simulink model "lab3_step3"  (R2019b)
settings: Solver=VariableStepAuto  StartTime=0.0  StopTime=stop_time  RelTol=1e-3
InitFcn:
  | %Read in the audio file
  | [input_wav_signal, Fs_in] = audioread('acoustic.wav');
  | % Fs_in = 11025 and we need to convert this to Fs = 48k
  | 
  | % COnvert the Sampling rate to 48 kHz
  | signal = resample(input_wav_signal, 48000, 11025);
  | Fs = 48000; % This is out desired sample rate that we converted to
  | Ts = 1/Fs;    % and the associated sample period.
  | 
  | % Put signal into a timeseries format
  | timevals = [0:length(signal)-1]*Ts;
  | input_signal = timeseries(signal,timevals);
  | 
  | % Set the simulation stop time
  | stop_time = length(signal) * Ts; % set the simulation time the same length as the input signal
  | 
  | 
  | % Fixed-point precision we want the signal converted to.
  | W_bits = 32;
  | F_bits = 28;
  | 
  | max_reset_Nsamples = 1024*16 % should be a power of 2
  | max_reset_Nbits = ceil (log2 (max_reset_Nsamples));
StopFcn:
  | y_out = output_signal.Data(:);
  | plot(y_out)
  | soundsc(y_out,Fs)
undefined symbols (not defined in the file): magnitude
libraries: simulink x2
settings Model: Creator=yassi  LastModifiedBy=yassi
settings DataIOCC: ReturnWorkspaceOutputs=off

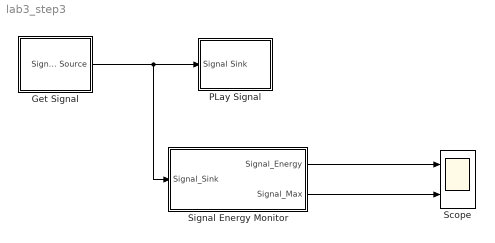
== system lab3_step3 ==
  Get Signal : Subsystem
  PLay Signal : Subsystem
  Scope : Scope  NumInputPorts=2
  Signal Energy Monitor : Subsystem
  wires:
  Get Signal/1(Signal Source) -> Signal Energy Monitor/1(Signal_Sink), PLay Signal/1(Signal Sink)
  Signal Energy Monitor/1(Signal_Energy) -> Scope/1
  Signal Energy Monitor/2(Signal_Max) -> Scope/2

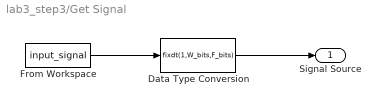
== system lab3_step3/Get Signal ==
  Data Type Conversion : DataTypeConversion  OutDataTypeStr=fixdt(1,W_bits,F_bits)
  From Workspace : FromWorkspace  VariableName=input_signal  SampleTime=Ts
  Signal Source : Outport
  wires:
  From Workspace/1 -> Data Type Conversion/1
  Data Type Conversion/1 -> Signal Source/1

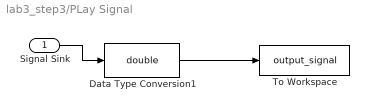
== system lab3_step3/PLay Signal ==
  Signal Sink : Inport
  Data Type Conversion1 : DataTypeConversion  OutDataTypeStr=double
  To Workspace : ToWorkspace  VariableName=output_signal  SaveFormat=Timeseries  SampleTime=-1
  wires:
  Data Type Conversion1/1 -> To Workspace/1
  Signal Sink/1 -> Data Type Conversion1/1

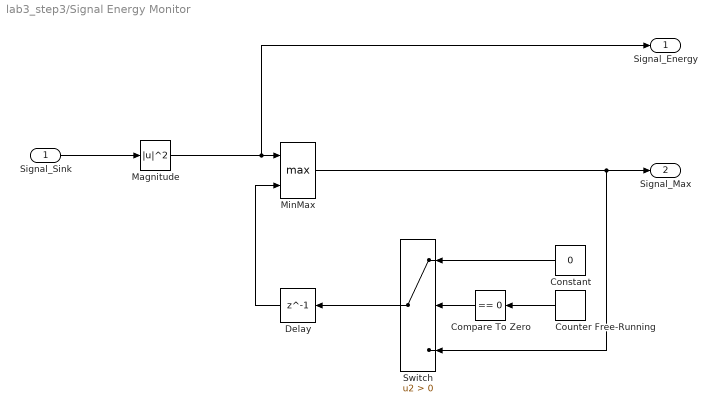
== system lab3_step3/Signal Energy Monitor ==
  Signal_Sink : Inport
  Compare To Zero : simulink/Logic and Bit Operations/Compare To Zero  relop===  OutDataTypeStr=boolean
  Constant : Constant  Value=0  OutDataTypeStr=fixdt(1,W_bits,F_bits)  SampleTime=Ts
  Counter Free-Running : simulink/Sources/Counter Free-Running  NumBits=max_reset_Nbits  tsamp=Ts
  Delay : Delay  DelayLength=1
  Magnitude : Math  Operator=magnitude^2  RndMeth=Zero  SaturateOnIntegerOverflow=on
  MinMax : MinMax  Function=max  Inputs=2
  Switch : Switch  Criteria=u2 > Threshold
  Signal_Energy : Outport
  Signal_Max : Outport  Port=2
  wires:
  Magnitude/1 -> Signal_Energy/1, MinMax/1
  MinMax/1 -> Switch/3, Signal_Max/1
  Delay/1 -> MinMax/2
  Signal_Sink/1 -> Magnitude/1
  Switch/1 -> Delay/1
  Constant/1 -> Switch/1
  Counter Free-Running/1 -> Compare To Zero/1
  Compare To Zero/1 -> Switch/2
